simulink model "DCMotor"  (R2024b)
settings: Solver=VariableStepAuto  StartTime=0.0  StopTime=0.6  RelTol=1e-3
InitFcn:
  | Vin = single(12);          %Armature voltage
  | 
  | Ra = single(2.461);        %armature resistance
  | La = single(0.0351);       %armature inductance
  | Rf = single(47.74);        %
  | Lf = single(0.3364);       %
  | KLm = single(0.1963);
  | If = single(Vin/Rf);
  | J = single(0.0138);        % Inertia moment
  | f = single(0.1);           % Viscous friction coefitient
  | Tm = 0;                    % Load torque Nm
  | 
  | overLa = 1/La;
  | overJ = 1/J;
  | K = KLm*If;
  | 
  | h = 4e-6;
settings Model: Creator=User  LastModifiedBy=User

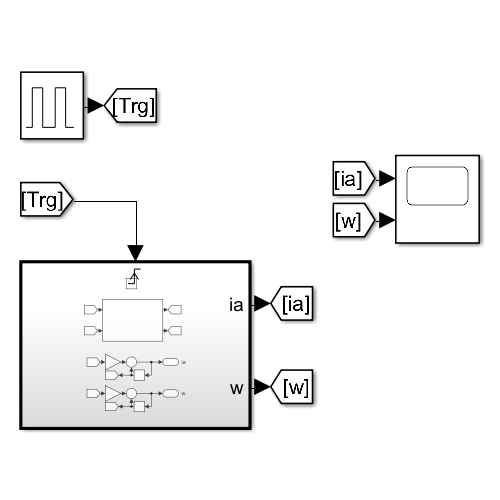
[thumbnail: Simulink's stored preview of the top-level diagram]
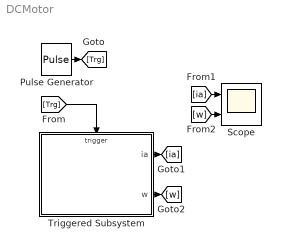
== system DCMotor ==
  Pulse Generator : DiscretePulseGenerator  PulseType=Time based  Period=h  PulseWidth=5
  Scope : Scope  NumInputPorts=2
  Triggered Subsystem : Subsystem  TreatAsAtomicUnit=on
  wires:
  Pulse Generator/1 -> [Trg]
  [Trg] -> Triggered Subsystem/Trigger
  Triggered Subsystem/1(ia) -> [ia]
  Triggered Subsystem/2(w) -> [w]
  [ia] -> Scope/1
  [w] -> Scope/2

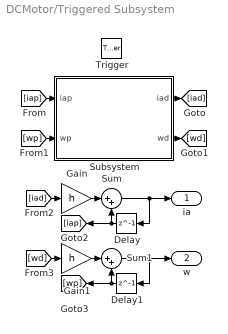
== system DCMotor/Triggered Subsystem ==
  Trigger : TriggerPort  VariantControl=(inherit)
  Delay : Delay  DelayLength=1
  Delay1 : Delay  DelayLength=1
  Gain : Gain  Gain=h
  Gain1 : Gain  Gain=h
  Subsystem : Subsystem
  Sum : Sum  Inputs=|++  OutDataTypeStr=single
  Sum1 : Sum  Inputs=|++  OutDataTypeStr=single
  ia : Outport
  w : Outport  Port=2
  wires:
  Sum/1 -> ia/1, Delay/1
  Subsystem/1(iad) -> [iad]
  Subsystem/2(wd) -> [wd]
  [iap] -> Subsystem/1(iap)
  [wp] -> Subsystem/2(wp)
  Gain/1 -> Sum/1
  [iad] -> Gain/1
  Delay/1 -> [iap], Sum/2
  Delay1/1 -> Sum1/2, [wp]
  Gain1/1 -> Sum1/1
  Sum1/1 -> w/1, Delay1/1
  [wd] -> Gain1/1

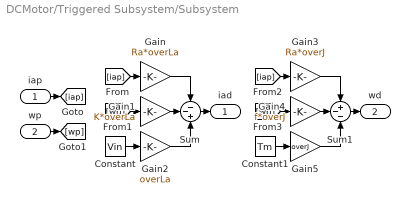
== system DCMotor/Triggered Subsystem/Subsystem ==
  iap : Inport
  wp : Inport  Port=2
  Constant : Constant  Value=Vin
  Constant1 : Constant  Value=Tm
  Gain : Gain  Gain=Ra*overLa
  Gain1 : Gain  Gain=K*overLa
  Gain2 : Gain  Gain=overLa
  Gain3 : Gain  Gain=Ra*overJ
  Gain4 : Gain  Gain=f*overJ
  Gain5 : Gain  Gain=overJ
  Sum : Sum  Inputs=--+  OutDataTypeStr=single
  Sum1 : Sum  Inputs=+--  OutDataTypeStr=single
  iad : Outport
  wd : Outport  Port=2
  wires:
  iap/1 -> [iap]
  wp/1 -> [wp]
  [iap] -> Gain/1
  Gain/1 -> Sum/1
  Gain1/1 -> Sum/2
  [wp] -> Gain1/1
  Constant/1 -> Gain2/1
  Gain2/1 -> Sum/3
  Sum/1 -> iad/1
  Sum1/1 -> wd/1
  Constant1/1 -> Gain5/1
  [wp] -> Gain4/1
  [iap] -> Gain3/1
  Gain4/1 -> Sum1/2
  Gain3/1 -> Sum1/1
  Gain5/1 -> Sum1/3
